simulink model "Part3_regulatory"  (R2021b)
settings: Solver=VariableStepAuto  StartTime=0.0  StopTime=20  RelTol=1e-6
libraries: slpidlib x1
settings Model: Creator=homan  LastModifiedBy=homan

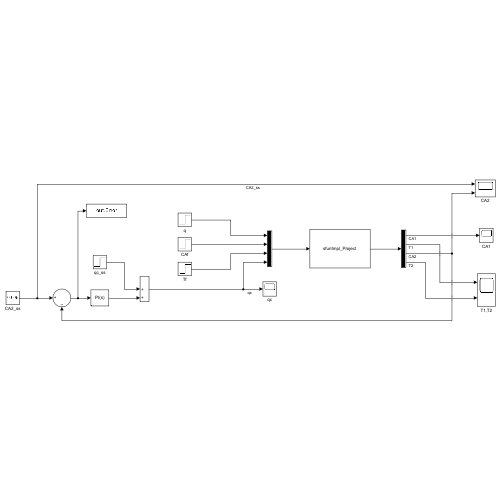
[thumbnail: Simulink's stored preview of the top-level diagram]
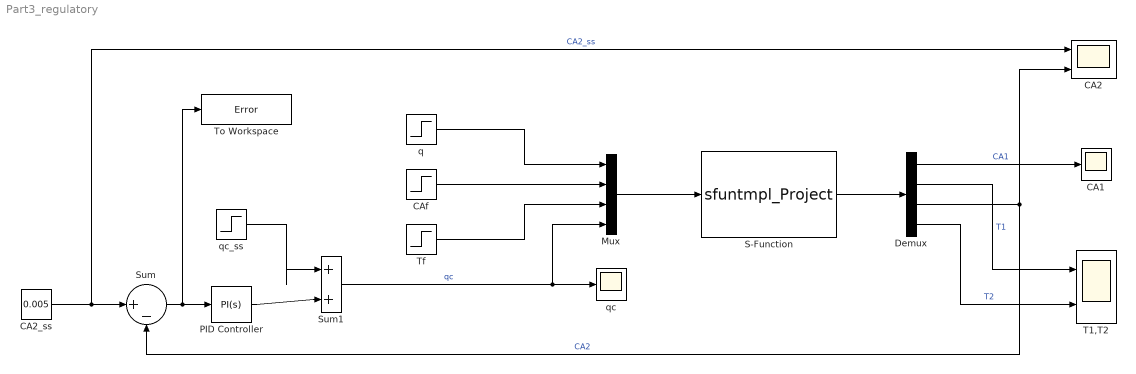
== system Part3_regulatory ==
  CA1 : Scope
  CA2 : Scope  NumInputPorts=2
  CA2_ss : Constant  Value=0.005
  CAf : Step  Time=5  Before=1  After=1*1.1  SampleTime=0
  Demux : Demux
  Mux : Mux
  PID Controller : slpidlib/PID Controller  Controller=PI  Form=Parallel  TimeDomain=Continuous-time  UseExternalTs=off  SampleTime=-1  IntegratorMethod=Forward Euler  FilterMethod=Forward Euler  ControllerParametersSource=internal  P=1831  I=6390  D=0  UseFilter=on  N=100  TunerSelectOption=Transfer Function Based (PID Tuner App)  InitialConditionSource=internal  InitialConditionForIntegrator=0  InitialConditionForFilter=0  DifferentiatorICPrevScaledInput=0  ExternalReset=none  TrackingMode=off  Kt=1  LimitOutput=off  SatLimitsSource=internal  UpperSaturationLimit=inf  LowerSaturationLimit=-inf  LinearizeAsGain=on  AntiWindupMode=none  Kb=1  POutMin=[]  POutMax=[]  IOutMin=[]  IOutMax=[]  DOutMin=[]  DOutMax=[]  NOutMin=[]  NOutMax=[]  SumOutMin=[]  SumOutMax=[]  SaturationOutMin=[]  SaturationOutMax=[]  PParamMin=[]  PParamMax=[]  IParamMin=[]  IParamMax=[]  DParamMin=[]  DParamMax=[]  NParamMin=[]  NParamMax=[]  KbParamMin=[]  KbParamMax=[]  KtParamMin=[]  KtParamMax=[]  KbOutMin=[]  KbOutMax=[]  KtOutMin=[]  KtOutMax=[]  IntegratorOutMin=[]  IntegratorOutMax=[]  FilterOutMin=[]  FilterOutMax=[]  SumI1OutMin=[]  SumI1OutMax=[]  SumI2OutMin=[]  SumI2OutMax=[]  SumI3OutMin=[]  SumI3OutMax=[]  SumI4OutMin=[]  SumI4OutMax=[]  SumDOutMin=[]  SumDOutMax=[]  DifferentiatorOutMin=[]  DifferentiatorOutMax=[]  FilterDiffOutCoefMin=[]  FilterDiffOutCoefMax=[]  ReciprocalOutMin=[]  ReciprocalOutMax=[]  SumDenOutMin=[]  SumDenOutMax=[]  SumNumOutMin=[]  SumNumOutMax=[]  DivideOutMin=[]  DivideOutMax=[]  UdiffTsProdOutMin=[]  UdiffTsProdOutMax=[]  NTsProdOutMin=[]  NTsProdOutMax=[]  UintegralTsProdOutMin=[]  UintegralTsProdOutMax=[]  UngainTsProdOutMin=[]  UngainTsProdOutMax=[]  IntegratorContinuousStateAttributes=''  IntegratorStateMustResolveToSignalObject=off  IntegratorRTWStateStorageClass=Auto  FilterContinuousStateAttributes=''  FilterStateMustResolveToSignalObject=off  FilterRTWStateStorageClass=Auto  ParallelPVariant=InternalParameters  IdealPVariant=Disabled  IVariant=InternalParameters  DVariant=Disabled  IntegratorVariant=Continuous  SatVariant=Disabled  AWVariant=Passthrough  PCopyVariant=Disabled  TRVariant=Disabled  FdbkBlocksVariant=Forward  IdealPFdbkVariant=Disabled  SatFdbkVariant=Disabled  DerivativeFilterVariant=Disabled  NVariant=Disabled  NCopyVariant=Disabled_SignalSpec  FilterICVariant=Disabled  IntegratorICVariant=InternalICs  ExternalResetVariant=Disabled  TRSumVariant=Passthrough  SumFdbkVariant=Disabled  SumVariant=Sum_PI  TsampFilterVariant=InternalTs  TsampNgainVariant=Passthrough  TsampIntegralVariant=Passthrough  ExternalSaturationOutDataTypeStr=Inherit: Same as second input
  S-Function : S-Function  FunctionName=sfuntmpl_Project  SFunctionDeploymentMode=off  EnableBusSupport=off
  Sum : Sum  Inputs=|+-
  Sum1 : Sum  Inputs=|++
  T1,T2 : Scope  NumInputPorts=2
  Tf : Step  Time=5  Before=350  After=350*1.1  SampleTime=0
  To Workspace : ToWorkspace  VariableName=Error  SaveFormat=Timeseries  SampleTime=-1
  q : Step  Time=5  Before=100  After=100*1.1  SampleTime=0
  qc : Scope
  qc_ss : Step  Time=5  Before=99  After=99*1.1  SampleTime=0
  wires:
  Demux/1 -> CA1/1  "CA1"
  Demux/4 -> T1,T2/2  "T2"
  Tf/1 -> Mux/3
  CA2_ss/1 -> CA2/1, Sum/1  "CA2_ss"
  Demux/2 -> T1,T2/1  "T1"
  Mux/1 -> S-Function/1
  Demux/3 -> Sum/2, CA2/2  "CA2"
  S-Function/1 -> Demux/1
  q/1 -> Mux/1
  CAf/1 -> Mux/2
  qc_ss/1 -> Sum1/1
  PID Controller/1 -> Sum1/2
  Sum/1 -> To Workspace/1, PID Controller/1
  Sum1/1 -> qc/1, Mux/4  "qc"
